simulink model "model"  (R2014b)
settings: Solver=ode45  StartTime=0.0  StopTime=40  MaxStep=0.01  RelTol=1e-3
values from neighbouring files (symbols this model uses):
  n = input(prompt)    [rander.m]
undefined symbols (not defined in the file or in its folder): adapt, K, sigma_0, vd, X, Y, zeta_0
settings Model: CovSFcnEnable=on  Creator=Marta_2805  LastModifiedBy=Demijan
settings SolverCC: AutoInsertRateTranBlk=on
settings OptimizationCC: UseDivisionForNetSlopeComputation=off  SimCompilerOptimization=off
settings DebuggingCC: UnderspecifiedInitializationDetection=Classic  MergeDetectMultiDrivingBlocksExec=none  FrameProcessingCompatibilityMsg=error
settings RTWCC: RTWCompilerOptimization=off

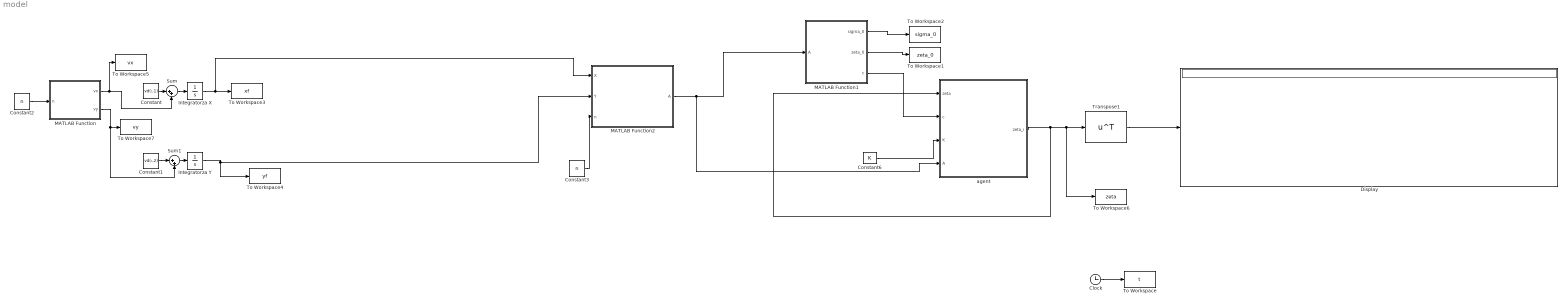
== system model ==
  Clock : Clock
  Constant : Constant  Value=vd(:,1)
  Constant1 : Constant  Value=vd(:,2)
  Constant2 : Constant  Value=n
  Constant3 : Constant  Value=n
  Constant6 : Constant  Value=K
  Display : Display
  Integratorza X : Integrator  InitialCondition=X  LimitOutput=on  UpperSaturationLimit=20  LowerSaturationLimit=0
  Integratorza Y : Integrator  InitialCondition=Y  LimitOutput=on  UpperSaturationLimit=20  LowerSaturationLimit=0
  MATLAB Function : MATLAB Function  TreatAsAtomicUnit=on
  MATLAB Function1 : MATLAB Function  TreatAsAtomicUnit=on
  MATLAB Function2 : MATLAB Function  TreatAsAtomicUnit=on
  Sum : Sum  Inputs=|++
  Sum1 : Sum  Inputs=|++
  To Workspace : ToWorkspace  VariableName=t  SampleTime=-1
  To Workspace1 : ToWorkspace  VariableName=zeta_0  SaveFormat=Structure  SampleTime=-1
  To Workspace2 : ToWorkspace  VariableName=sigma_0  SaveFormat=Structure  SampleTime=-1
  To Workspace3 : ToWorkspace  VariableName=xf  SaveFormat=Structure  SampleTime=-1
  To Workspace4 : ToWorkspace  VariableName=yf  SaveFormat=Structure  SampleTime=-1
  To Workspace5 : ToWorkspace  VariableName=vx  SaveFormat=Structure  SampleTime=-1
  To Workspace6 : ToWorkspace  VariableName=zeta  SampleTime=-1
  To Workspace7 : ToWorkspace  VariableName=vy  SaveFormat=Structure  SampleTime=-1
  Transpose1 : Math  Operator=transpose  SaturateOnIntegerOverflow=on
  "agent " : Subsystem
  wires:
  Constant6/1 -> "agent "/3(K)
  MATLAB Function1/3(c) -> "agent "/2(c)
  "agent "/1(zeta_i) -> "agent "/1(zeta), To Workspace6/1, Transpose1/1
  Transpose1/1 -> Display/1
  Clock/1 -> To Workspace/1
  MATLAB Function1/2(zeta_0) -> To Workspace1/1
  MATLAB Function1/1(sigma_0) -> To Workspace2/1
  Integratorza Y/1 -> MATLAB Function2/2(Y), To Workspace4/1
  Integratorza X/1 -> MATLAB Function2/1(X), To Workspace3/1
  Constant/1 -> Sum/1
  Sum/1 -> Integratorza X/1
  Constant1/1 -> Sum1/1
  Sum1/1 -> Integratorza Y/1
  Constant2/1 -> MATLAB Function/1(n)
  MATLAB Function/1(vx) -> To Workspace5/1, Sum/2
  MATLAB Function/2(vy) -> To Workspace7/1, Sum1/2
  Constant3/1 -> MATLAB Function2/3(n)
  MATLAB Function2/1(A) -> "agent "/4(A), MATLAB Function1/1(A)

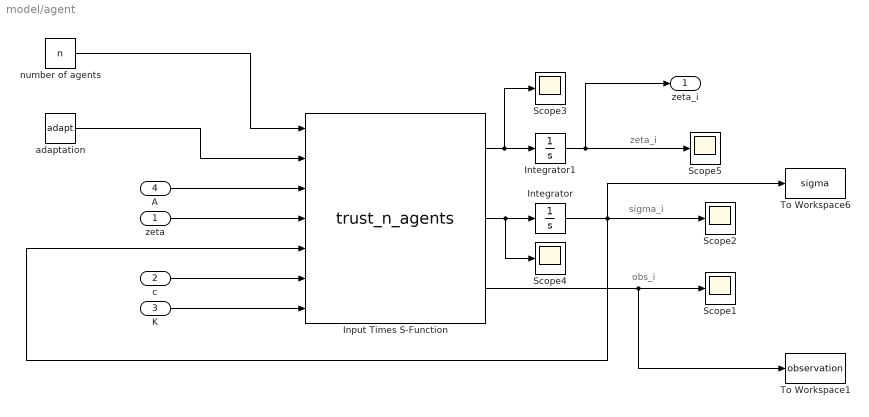
== system model/agent  ==
  note: obs_i
  note: sigma_i
  note: zeta_i
  zeta : Inport
  c : Inport  Port=2
  K : Inport  Port=3
  A : Inport  Port=4
  Input Times S-Function : S-Function  FunctionName=trust_n_agents  EnableBusSupport=off
  Integrator : Integrator  InitialCondition=sigma_0
  Integrator1 : Integrator  InitialCondition=zeta_0
  Scope{1..5} (5 alike) : Scope
      Scope1 settings: TimeRange=20  YMin=0.25  YMax=0.95
      Scope2 settings: TimeRange=20  YMin=0.25  YMax=0.95
      Scope3 settings: TimeRange=20  YMin=0.25  YMax=0.95  SaveName=ScopeData3
      Scope4 settings: TimeRange=20  YMin=0.25  YMax=0.95  SaveName=ScopeData4
      Scope5 settings: TimeRange=20  YMin=0.25  YMax=0.95  SaveName=ScopeData2
  To Workspace1 : ToWorkspace  VariableName=observation  SampleTime=-1
  To Workspace6 : ToWorkspace  VariableName=sigma  SampleTime=-1
  adaptation : Constant  Value=adapt
  number of agents : Constant  Value=n
  zeta_i : Outport
  wires:
  Integrator/1 -> Scope2/1, Input Times S-Function/5, To Workspace6/1
  Integrator1/1 -> zeta_i/1, Scope5/1
  c/1 -> Input Times S-Function/6
  K/1 -> Input Times S-Function/7
  Input Times S-Function/2 -> Scope4/1, Integrator/1
  Input Times S-Function/1 -> Scope3/1, Integrator1/1
  Input Times S-Function/3 -> To Workspace1/1, Scope1/1
  number of agents/1 -> Input Times S-Function/1
  adaptation/1 -> Input Times S-Function/2
  A/1 -> Input Times S-Function/3
  zeta/1 -> Input Times S-Function/4

== matlab function model/MATLAB Function1 ==
  data: A input; sigma_0 output; zeta_0 output; c output
function [sigma_0, zeta_0, c] = fcn(A)

sigma_0 = zeros(20,20);
c = zeros(20,20);

  for i=1:n 
    delta = roundn(rand(),-1);
    for j=1:n
        if A(j,i) == 1
            sigma_0(j,i) = roundn(rand(),-1);    
            c(j,i) = delta;
        end
    end
  end


%check a spanning tree
deg = diag(sum(A,2));
L = deg - A;
row_sum = sum (L,2);

%V - full matrix whose columns are the corresponding eigenvectors
%D - diagonal matrix D of eigenvalues
[V, D] = eig(L);
D = diag(D);
D = floor(D);

number = size((find(D == 0)),1);     %number of eigenvalues = 0
if (number == 1)
    pr = round(L * V(:,find(D==0)));
end

if (row_sum == 0 & pr == 0 & number == 1) 
    flag = 0;
end

== matlab function model/MATLAB Function ==
  settings: updateMethod=DISCRETE  sampleTime=0.01
  data: vx output size=20 [-5..5]; vy output size=20 [-5..5]; n input
function [vx, vy] = fish(n)
vx=zeros(20,1);
vy=zeros(20,1);
for i=1:n;
    vx(i)=4*(rand-0.5);
    vy(i)=4*(rand-0.5);
end

== matlab function model/MATLAB Function2 ==
  settings: updateMethod=DISCRETE  sampleTime=0.01
  data: X input; Y input; n input; A output
function A  = fish(X, Y, n)
A=zeros(20,20);
for i=1:n;
    for j=1:n;
        R = sqrt(((X(i)-X(j))^2+(Y(i)-Y(j))^2));
        if R < 4 && i~=j;
            A(i,j)=1;
        else
            A(i,j)=0;
        end
    end
end
